simulink model "MotoShield_Compensator"  (R2019a)
settings: Solver=FixedStepAuto  StartTime=0.0  StopTime=20  RelTol=1e-3  EnableMultiTasking=on
libraries: MotoLibrary x2, CommonBlocks x1, simulink x1
settings Model: ExtModeTrigDuration=2  Creator=JB  LastModifiedBy=JB
settings OptimizationCC: EnhancedBackFolding=on  PassReuseOutputArgsThreshold=0  MaxStackSize=64  OptimizeBlockOrder=speed  DifferentSizesBufferReuse=on  OptimizationCustomize=off
settings DebuggingCC: ParameterTunabilityLossMsg=error
settings HardwareCC: ProdBitPerInt=16  ProdBitPerPointer=16  ProdBitPerSizeT=16  ProdBitPerPtrDiffT=16  ProdLargestAtomicFloat=None  ProdWordSize=8  ProdHWDeviceType=Atmel->AVR  UseEmbeddedCoderFeatures=off  UseSimulinkCoderFeatures=off
settings SFSimCC: MATLABDynamicMemAlloc=off
settings RTWCC: SystemTargetFile=ert.tlc  HardwareBoard=Arduino Uno  TLCOptions=-aInlineSetEventsForThisBaseRateFcn=TLC_FALSE -aSuppressMultiTaskScheduler=TLC_FALSE -aRateBasedStepFcn=1  TemplateMakefile=ert_default_tmf  GenerateReport=on  Toolchain=Arduino AVR  BuildConfiguration=Faster Runs  LaunchReport=on
settings CodeAppCC: ForceParamTrailComments=on  OperatorAnnotations=on
settings ERTTargetCC: ERTCustomFileBanners=off  SupportContinuousTime=on  SupportNonInlinedSFcns=on  RemoveResetFunc=off  SupportVariableSizeSignals=on  ModelStepFunctionPrototypeControlCompliant=off  ExtModeStaticAllocSize=250

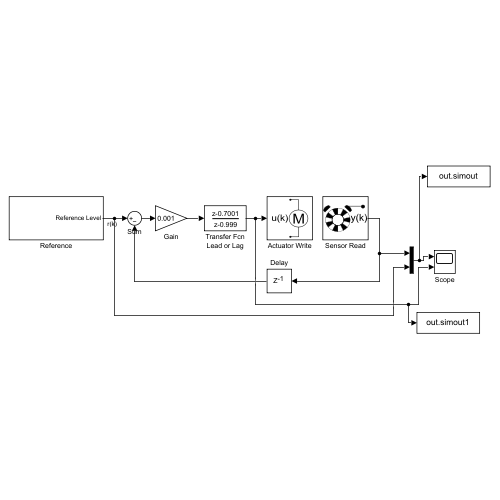
[thumbnail: Simulink's stored preview of the top-level diagram]
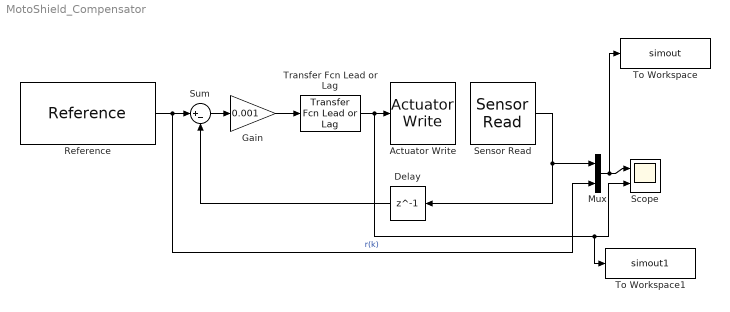
== system MotoShield_Compensator ==
  Actuator Write : MotoLibrary/Actuator Write  ShieldRelease=R2  inputType=Voltage (V)  dir=Clockwise
  Delay : Delay  DelayLength=1
  Gain : Gain  Gain=0.001
  Mux : Mux  Inputs=2
  Reference : CommonBlocks/Reference  RefVect=[1200.0,800.0,1200.0,1000.0,700.0,1000.0,1200.0,600.0,1100.0,500.0,0.0]  AtTheEnd=Stop simulation  Reps=5  SectLen=100  OffsetTime=0  Ts=0.02
      settings: SourceProductName=AutomationShield
  Scope : Scope  NumInputPorts=2
  Sensor Read : MotoLibrary/Sensor Read  ShieldRelease=R2  outputType=Radian per second (rad/s)  calibrationValues=Use default values  minValue=800  maxValue=2060  Ts=0.02
      link override SensorReadR2/Gain5: Gain=1/28
  Sum : Sum  Inputs=|+-
  To Workspace : ToWorkspace  VariableName=simout  SampleTime=-1
  To Workspace1 : ToWorkspace  VariableName=simout1  SampleTime=-1
      settings: Save2DSignal=2-D array (concatenate along first dimension)
  Transfer Fcn Lead or Lag : simulink/Discrete/Transfer Fcn Lead or Lag  PoleZ=0.999  ZeroZ=0.7001  ICPrevOutput=0.0  ICPrevInput=0.0  RndMeth=Ceiling  DoSatur=on
      settings: SourceProductBaseCode=SL
  wires:
  Sensor Read/1 -> Mux/1, Delay/1
  Delay/1 -> Sum/2
  Reference/1 -> Mux/2, Sum/1  "r(k)"
  Transfer Fcn Lead or Lag/1 -> To Workspace1/1, Scope/2, Actuator Write/1
  Sum/1 -> Gain/1
  Gain/1 -> Transfer Fcn Lead or Lag/1
  Mux/1 -> To Workspace/1, Scope/1
